simulink model "rpi_button_A_B"  (R2017a)
settings: Solver=VariableStepAuto  StartTime=0.0  StopTime=inf  RelTol=1e-3
undefined symbols (not defined in the file): Green, led0
libraries: embdlinuxlib x3
settings Model: SimulationMode=external  Creator=WARA  LastModifiedBy=WARA

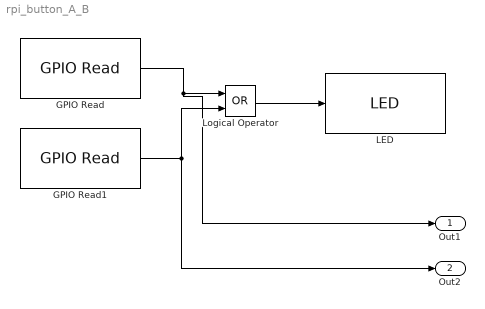
== system rpi_button_A_B ==
  GPIO Read : embdlinuxlib/GPIO Read  board=Pi 3 Model B  gpio=22  internalResistor=Off  sampleTime=0.1  direction=Input  blockPlatform=Raspberry Pi
  GPIO Read1 : embdlinuxlib/GPIO Read  board=Pi 3 Model B  gpio=27  internalResistor=Off  sampleTime=0.1  direction=Input  blockPlatform=Raspberry Pi
  LED : embdlinuxlib/LED  board=Pi 2 Model B  led=led0 (Green)  blockPlatform=Raspberry Pi
  Logical Operator : Logic  Operator=OR  AllPortsSameDT=off  OutDataTypeStr=boolean
  Out1 : Outport
  Out2 : Outport  Port=2
  wires:
  Logical Operator/1 -> LED/1
  GPIO Read/1 -> Out1/1, Logical Operator/1
  GPIO Read1/1 -> Out2/1, Logical Operator/2
